simulink model "JenaFox_NCm"  (R2022a)
settings: Solver=VariableStepAuto  StartTime=0.0  StopTime=terminationConditions.stopTime  FixedStep=0.0001  MaxStep=solverParams.maxStep  RelTol=solverParams.relTol  AbsTol=solverParams.absTol
undefined symbols (not defined in the file): amplifier, c_coupling, d_coupling, g, GC, GM_h, IC, IC_v, motorHip, motorKnee, mu, offset, prop_const, smiData, terminationConditions, v, X, Y, Z
libraries: sm_lib x51, nesl_utility x46, simulink x23, simulink_extras x12, dspswit3 x2
(part 4 of 4)

== system JenaFox_NCm/JenaFox Model/GCM Right/Ground Friction Model/X-Axis Kinetic Friction Model ==
  note: Kinetic Friction Model
  note: Footpoint Determiner
  note: Sliding Limit Detector
  pos [m] : Inport
  vel [m/s] : Inport  Port=2
  F_Normal [N] : Inport  Port=3
  Enable : EnablePort  StatesWhenEnabling=reset  PropagateVarSize=During execution
  Abs : Abs  SaturateOnIntegerOverflow=off
  Constant : Constant  Value=v.limit
  FixPt Relational Operator : RelationalOperator  Operator=>  OutDataTypeStr=boolean  ZeroCross=off  InputSameDT=off
  Memory : Memory  InheritSampleTime=on
  Negative : simulink/Logic and Bit Operations/Compare To Zero  relop=<  OutDataTypeStr=boolean
  Product : Product  RndMeth=Zero
  Sign1 : Signum
  Sum : Sum  Inputs=|+-
  reverse : Gain  Gain=-1
  sliding friction coefficient : Gain  Gain=mu.slide
  posFP [m] : Outport  VectorParamsAs1DForOutWhenUnconnected=off
      settings: AttributesFormatString=initial = '%<InitialOutput>'\nwhen disabled = '%<OutputWhenDisabled>'
  Stiction! : Outport  Port=2  OutputWhenDisabled=reset  InitialOutput=0  VectorParamsAs1DForOutWhenUnconnected=off
      settings: AttributesFormatString=initial = '%<InitialOutput>'\nwhen disabled = '%<OutputWhenDisabled>'
  F_Slide [N] : Outport  Port=3  OutputWhenDisabled=reset  InitialOutput=0  VectorParamsAs1DForOutWhenUnconnected=off
      settings: AttributesFormatString=initial = '%<InitialOutput>'\nwhen disabled = '%<OutputWhenDisabled>'
  wires:
  reverse/1 -> Product/1
  F_Normal [N]/1 -> sliding friction coefficient/1
  vel [m/s]/1 -> Sign1/1, Abs/1
  pos [m]/1 -> posFP [m]/1
  Product/1 -> F_Slide [N]/1
  sliding friction coefficient/1 -> Product/2
  Sign1/1 -> reverse/1
  Memory/1 -> FixPt Relational Operator/2
  Negative/1 -> Memory/1, FixPt Relational Operator/1
  Abs/1 -> Sum/1
  Sum/1 -> Negative/1
  Constant/1 -> Sum/2
  FixPt Relational Operator/1 -> Stiction!/1

== system JenaFox_NCm/JenaFox Model/GCM Right/Ground Friction Model/X-Axis Static Friction Model ==
  note: Stiction Limit Detector
  note: Static Friction Model
  note: Zero multiplication prevents
      | horizontal friction model from
      | oscillating between static and kinetic
      | friction when the vertical force is zero but
      | the ground level is not yet reached
      | in the upward motion
  F_Normal [N] : Inport
  pos [m] : Inport  Port=2
  vel [m/s] : Inport  Port=3
  posFP [m] : Inport  Port=4
  Enable : EnablePort  StatesWhenEnabling=reset  PropagateVarSize=During execution
  Abs : Abs  SaturateOnIntegerOverflow=off
  Abs. : Abs  SaturateOnIntegerOverflow=off
  Check Vertical Friction : Product  RndMeth=Zero
  FixPt Relational Operator : RelationalOperator  Operator=>  OutDataTypeStr=boolean  ZeroCross=off  InputSameDT=off
  Gain3 : Gain  Gain=GC.k_gx
  Gain4 : Gain  Gain=1/v.gx_max
  Memory : Memory
  Mux1 : Mux  Inputs=2
  Positive : simulink/Logic and Bit Operations/Compare To Zero  relop=>  OutDataTypeStr=boolean
  Positive1 : simulink/Logic and Bit Operations/Compare To Zero  relop=>  OutDataTypeStr=boolean
  Sum : Sum  Inputs=-+
  Sum2 : Sum  Inputs=-+|
  X-Axis Stiction Force2 : Fcn  Expr=-u(1) * (1+sgn(u(1))*u(2)) * ( (1+sgn(u(1))*u(2))>0)
  stiction limit force : Gain  Gain=mu.stick
  F_Stick [N] : Outport  OutputWhenDisabled=reset  InitialOutput=0  VectorParamsAs1DForOutWhenUnconnected=off
      settings: AttributesFormatString=when disabled: %<OutputWhenDisabled>\ninitial: %<InitialOutput>
  Sliding! : Outport  Port=2  OutputWhenDisabled=reset  InitialOutput=0  VectorParamsAs1DForOutWhenUnconnected=off
      settings: AttributesFormatString=when disabled: %<OutputWhenDisabled>\ninitial: %<InitialOutput>
  wires:
  F_Normal [N]/1 -> stiction limit force/1, Positive1/1
  Sum2/1 -> Gain3/1  "dx"
  pos [m]/1 -> Sum2/2
  posFP [m]/1 -> Sum2/1
  vel [m/s]/1 -> Gain4/1
  Sum/1 -> Positive/1
  Memory/1 -> FixPt Relational Operator/2
  Positive/1 -> FixPt Relational Operator/1, Memory/1
  Abs./1 -> Sum/2
  Mux1/1 -> X-Axis Stiction Force2/1
  Gain3/1 -> Mux1/1
  Gain4/1 -> Mux1/2
  FixPt Relational Operator/1 -> Sliding!/1
  Abs/1 -> Sum/1
  stiction limit force/1 -> Abs/1
  Positive1/1 -> Check Vertical Friction/2
  Check Vertical Friction/1 -> F_Stick [N]/1, Abs./1
  X-Axis Stiction Force2/1 -> Check Vertical Friction/1

== matlab function JenaFox_NCm/Touchdown/Calculate Angle of Attack1 ==
  data: alpha output; toe_r input; knee_r input
function alpha  = ...
    calc_angle_of_attack(toe_r, knee_r)

shank_r = knee_r - toe_r;
shank_r_x = dot(shank_r, [1; 0]);

alpha = acosd(norm(shank_r_x) / norm(shank_r));

end

== matlab function JenaFox_NCm/Mechanical Cost Analysis (MCA) (Lee, 2011)/Mechanical Cost Analysis (MCA) ==
  data: theta_com output; lambda_com output; lambda_hip output; lambda_proj output; phi_com output; V_proj output; AEA output; GRF input; origin_com input; V_com input; vphi_com input; origin_hip input; V_hip input; prop_const input; offset input
function [theta_com, lambda_com, lambda_hip, lambda_proj, phi_com, ...
    V_proj, AEA] = ... % , orbital_v_com, orbital_v_hip
    mechanical_cost_analysis(GRF, origin_com, V_com, vphi_com, origin_hip, V_hip, prop_const, offset) % , toe_r, vphi_hip, prop_const
% Mechanical cost analysis (method described in Lee 2011)


%% Instantaneous force angle ((Lee, 2011): equation 2)
Fy = norm(GRF(2));
F_norm = norm(GRF);
theta_com = acos(Fy / F_norm);
% theta_com = atan2(GRF(2), GRF(1));


%% Instantaneous velocity angle (CoM) ((Lee, 2011): equation 4)
Vx_com = norm(V_com(1));
V_norm_com = norm(V_com);
lambda_com = acos(Vx_com / V_norm_com);
% lambda_com = atan2(V_com(2), V_com(1));


%% Instantaneous velocity angle (hip) ((Lee, 2011): equation 4)
% Vx_hip = V_hip(1);
% % Vy_hip = V_hip(2);
% V_norm_hip = norm(V_hip);
% lambda_hip_cos = acos(Vx_hip / V_norm_hip);
% % lambda_hip = acosd(Vy_hip / V_norm_hip);
% % lambda_hip = atan2d(V_hip(2), V_hip(1));
lambda_hip = atan2(V_hip(2), V_hip(1));


%% Instantaneous velocity angle (CoM shifted to hip) ((Lee, 2011): equation 4)
angular_vel = cross([0; 0; vphi_com], [(origin_hip - origin_com); 0]);
V_proj = V_com + angular_vel(1:end - 1);
% Vx_proj = V_proj(1);
% % Vy_proj = abs(V_proj(2));
% V_norm_proj = norm(V_proj);
% lambda_proj_cos = acos(Vx_proj / V_norm_proj);
% % lambda_proj = acosd(Vy_proj / V_norm_proj);
lambda_proj = atan2d(V_proj(2), V_proj(1));

% AEA = lambda_proj - offset;
% AEA = -0.2 * lambda_proj - 25;
% AEA = 2 * lambda_proj - 45;
% AEA = 2.5 * lambda_proj - 75;
% AEA = 1.83 * lambda_proj - 80;
% AEA = prop_const * lambda_proj - offset;

% AEA = -0.015 * (lambda_proj ^ 2) - 10;

% AEA = -200 / lambda_proj;
% AEA = (-200 / lambda_proj) - 6;
% AEA = (-500 / lambda_proj) + 2;

% AEA = ((-prop_const / lambda_proj) - offset);
% AEA = (23 * (lambda_proj - 25) / lambda_proj) - offset;
% AEA = (37.6 / sqrt(2 * pi)) * exp(-0.002 * lambda_proj^2 / 2) - 25;

% AEA = ( -15 / (1 + exp(-0.3 * lambda_proj + 7))) - 10;
% AEA = ( -15 / (1 + exp(prop_const * lambda_proj + offset))) - 10;
AEA = ( 15 / (1 + exp(prop_const * lambda_proj + offset))) - 25;


% orbital_v_hip_full = cross([0; 0; vphi_hip], [(origin_hip - toe_r); 0]);
% orbital_v_hip  = orbital_v_hip_full(1:end - 1);
% 
% orbital_v_com_full  = cross([0; 0; vphi_com], [(origin_hip - toe_r); 0]);
% orbital_v_com = orbital_v_com_full(1:end - 1);


%% Angle between thigh and projected velocity vector
% thigh_r = origin_knee_r - origin_hip;
% rho = acosd( dot(thigh_r, V_proj) / (norm(thigh_r) * norm(V_proj)) );


%% Instantaneous collision angle ((Lee, 2011): equation 6)
% arcsin: represents phase shift of pi/2 to defone an angle of zero when F
% is perpendicular to V so that phi is directly proportional to the
% collision

% Limit value of input to the range [-1, 1] due to numerical issues
% phi_com = asin(max(min(norm(dot(GRF, V_com)) / ...
%     (norm(GRF) * norm(V_com)), 1), -1));
phi_com = asin(norm(dot(GRF, V_com)) / (norm(GRF) * norm(V_com)));
% phi_com = acos(norm(dot(GRF, V_com)) / (norm(GRF) * norm(V_com)));

end

== matlab function JenaFox_NCm/Neural Controller/Neural Network Based Controller ==
  data: t input; U output; phi input; GC input; AEA input; GM_h input; y_old input; y_old output
function [U, y_old] = neural_controller(t, phi, GC, AEA, GM_h, y_old)

%% controller settings
phi = phi';

t_old = y_old(1,1);
yFh_old = y_old(2,:);
yEh_old = y_old(3,:);
yFk_old = y_old(4,:);
yEk_old = y_old(5,:);

tau = 0.01;     % [s] time constant
alpha = 2;      % [1] response constant
Phi_Eh = 5;     % [deg] threshold sensor neuron hip extension, figure 5
Phi_Fh = AEA;   % -10; %[deg] threshold sensor neuron hip flexion
Phi_AL = Phi_Fh;
Phi_AR = Phi_Fh;
Phi_Ek = -4.25;
Phi_Fk = -80;
Phi_GL = 0.2;
Phi_GR = 0.2;
Phi_M = 1;    % bias firing treshold
M_Amp = 3;
% GM_h = 1.5;
GM_k = 0.9 * GM_h;
s_emh = 1;
s_fmh = -1;
s_emk = 1;
s_fmk = -1;

%% sensor neurons

%hip stretch receptors AL/AR, indicates when AEA is reached (hip flexed)
rho_AL = neuron(alpha,phi(2),Phi_AL);
rho_AR = neuron(alpha,phi(1),Phi_AR);

%ground contact sensors
rho_GL = neuron(alpha,Phi_GL,GC(2)-GC(1));
rho_GR = neuron(alpha,Phi_GR,GC(1)-GC(2));

% joint angle sensors hip
rho_Eh = neuron(alpha,Phi_Eh,phi(1:2));
rho_Fh = neuron(alpha,phi(1:2),Phi_Fh);

% joint angle sensors knee
rho_Ek = neuron(alpha,Phi_Ek,phi(3:4));
rho_Fk = neuron(alpha,phi(3:4),Phi_Fk);

%% motor neurons

%hip motor neurons
yEh = yEh_old * exp(-(t-t_old)/tau) + (-30) .* rho_Eh + [10 -10] .* rho_GR + [-10 10] .* rho_GL;
yFh = yFh_old * exp(-(t-t_old)/tau) + (-30) .* rho_Fh + [-10 10] .* rho_GR + [10 -10] .* rho_GL;

uEh = 1./(1 + exp(Phi_M-yEh));
uFh = 1./(1 + exp(Phi_M-yFh));

%knee motor neurons
yEk = yEk_old * exp(-(t-t_old)/tau) + (-30) .* rho_Ek + 15 .* [rho_AR rho_AL] + [10 -10] .* rho_GR + [-10 10] .* rho_GL;
yFk = yFk_old * exp(-(t-t_old)/tau) + (-30) .* rho_Fk + (-15) .* [rho_AR rho_AL] + [-10 10] .* rho_GR + [10 -10] .* rho_GL;

uEk = 1./(1 + exp(Phi_M-yEk));
uFk = 1./(1 + exp(Phi_M-yFk));

U = [M_Amp * GM_h .* (s_emh .* uEh + s_fmh .* uFh), M_Amp * GM_k .* (s_emk .* uEk + s_fmk .* uFk)]';

y_old(1,:) = [t 0];
y_old(3,:) = yEh;
y_old(2,:) = yFh;
y_old(5,:) = yEk;
y_old(4,:) = yFk;

    function rho = neuron(alpha,Phi_d,phi)
        rho = 1./(1 + exp(alpha .* (Phi_d - phi)));
    end

end
